simulink model "DC Dynamic Indhu Kanth"  (R2013a)
settings: Solver=ode45  StartTime=0.0  StopTime=2  RelTol=1e-3
libraries: powerlib x14, powerlib_extras x5, simulink x1
settings Model: Creator=Indhu Kanth  LastModifiedBy=Indhu Kanth

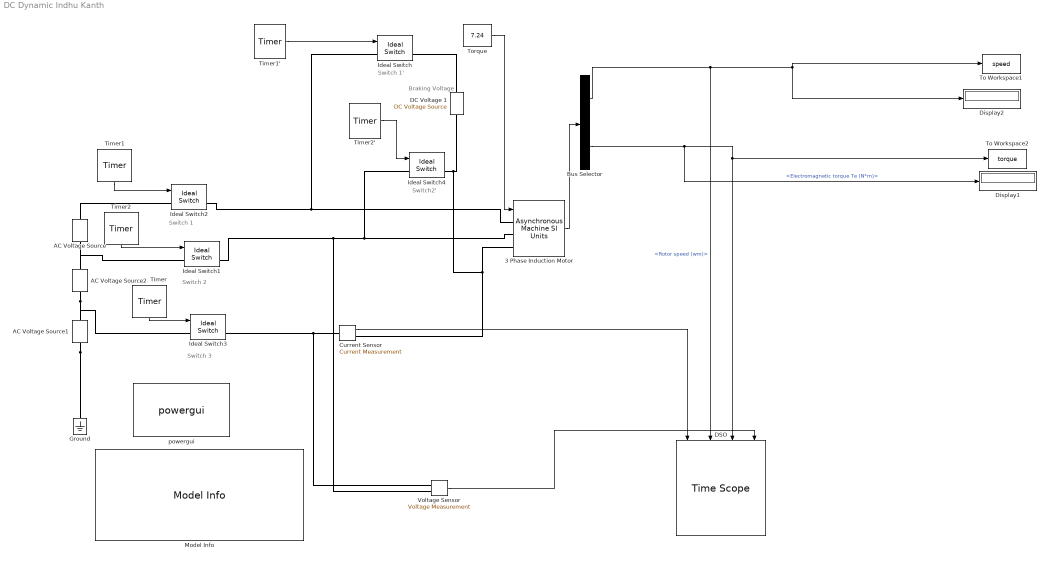
== system DC Dynamic Indhu Kanth ==
  note: Braking Voltage
  note: Switch2'
  note: Switch 1'
  note: Switch 3
  note: Switch 2
  note: Switch 1
  3 Phase Induction Motor : powerlib/Machines/Asynchronous Machine SI Units  PresetModel=No  MechanicalLoad=Torque Tm  ShowDetailedParameters=on  RotorType=Squirrel-cage  ReferenceFrame=Rotor  NominalParameters=[4427 440 50]  Stator="[0.5  0.003819]"  Rotor=[0.4 0.003819]  Cage1=[ 0.022 0.226/377]  Cage2=[ 0.022 0.226/377]  Lm=0.1591  Mechanical=[0.37 0.02791 3]  PolePairs=3  InitialConditions=[1 0 0 0 0 0 0 0]  Units=SI  LoadFlowParameters=1492000  SimulateSaturation=off  Saturation=[14.03593122, 27.81365428, 53.79336849, 72.68890987, 97.98006896, 148.6815601, 215.7428561, 302.9841135, 428.7778367 ; 230, 322, 414, 460, 506, 552, 598, 644, 690]  TsPowergui=0  TsBlock=-1  IterativeModel=Forward Euler  Pmec=0
  AC Voltage Source : powerlib/Electrical Sources/AC Voltage Source  Amplitude=230*sqrt(2)  Phase=0  Frequency=50  SampleTime=0  Measurements=None
  AC Voltage Source1 : powerlib/Electrical Sources/AC Voltage Source  Amplitude=230*sqrt(2)  Phase=120  Frequency=50  SampleTime=0  Measurements=None
  AC Voltage Source2 : powerlib/Electrical Sources/AC Voltage Source  Amplitude=230*sqrt(2)  Phase=-120  Frequency=50  SampleTime=0  Measurements=None
  Bus Selector : BusSelector  OutputSignals=Mechanical.Rotor speed (wm),Mechanical.Electromagnetic torque Te (N*m)
  Current Sensor : powerlib/Measurements/Current Measurement  PhasorSimulation=off  OutputType=Complex  PSBequivalent=0
  DC Voltage 1 : powerlib/Electrical Sources/DC Voltage Source  Amplitude=40  Measurements=None
  DSO : TimeScope  NumInputPorts=4  DefaultConfigurationName=spbscopes.TimeScopeBlockCfg
      settings: CopyFcn=scopeextensions.ScopeBlock.callback(gcbh, 'onBlockCopy', gcbh);  DeleteFcn=scopeextensions.ScopeBlock.callback(gcbh, 'onBlockDelete');  PreSaveFcn=scopeextensions.ScopeBlock.callback(gcbh, 'onModelSave');  NameChangeFcn=scopeextensions.ScopeBlock.callback(gcbh, 'onBlockRename');  CloseFcn=scopeextensions.ScopeBlock.callback(gcbh, 'onBlockClose');  PreDeleteFcn=scopeextensions.ScopeBlock.callback(gcbh, 'onBlockPreDelete');
  Display1 : Display
  Display2 : Display
  Ground : powerlib/Elements/Ground  LConnTagsString=a
  Ideal Switch : powerlib/Power Electronics/Ideal Switch  Ron=0.001  Lon=0  IC=0  Rs=1e5  Cs=inf  Measurements=on
  Ideal Switch1 : powerlib/Power Electronics/Ideal Switch  Ron=0.001  Lon=0  IC=1  Rs=1e5  Cs=inf  Measurements=on
  Ideal Switch2 : powerlib/Power Electronics/Ideal Switch  Ron=0.001  Lon=0  IC=1  Rs=1e5  Cs=inf  Measurements=on
  Ideal Switch3 : powerlib/Power Electronics/Ideal Switch  Ron=0.001  Lon=0  IC=1  Rs=1e5  Cs=inf  Measurements=on
  Ideal Switch4 : powerlib/Power Electronics/Ideal Switch  Ron=0.001  Lon=0  IC=0  Rs=1e5  Cs=inf  Measurements=on
  Model Info : simulink/Model-Wide Utilities/Model Info  InitialBlockCM=None  BlockCM=None  Frame=on  DisplayStringWithTags=|  HorizontalTextAlignment=Center  LeftAlignmentValue=0.5  SourceBlockDiagram=selfstudy1dcdynamic  TagMaxNumber=20
      | 3 PHASE INDUCTION MOTOR
      | DC Dynamic Braking
      | Indhy Kanth
  Timer : powerlib_extras/Control  Blocks/Timer  t=[0 0.5]  e="[1  0   ]"
  Timer1 : powerlib_extras/Control  Blocks/Timer  t=[0 0.5 ]  e="[1  0   ]"
  Timer1' : powerlib_extras/Control  Blocks/Timer  t=[0.5 1 ]  e=[1 1 ]
  Timer2 : powerlib_extras/Control  Blocks/Timer  t=[0 0.5 ]  e="[1  0   ]"
  Timer2' : powerlib_extras/Control  Blocks/Timer  t=[0.5 1]  e=[1 1 ]
  To Workspace1 : ToWorkspace  VariableName=speed  SampleTime=-1
  To Workspace2 : ToWorkspace  VariableName=torque  SampleTime=-1
  Torque : Constant  Value=7.24
  Voltage Sensor : powerlib/Measurements/Voltage Measurement  PhasorSimulation=off  OutputType=Complex  PSBequivalent=0
  powergui : powerlib/powergui  Priority=1  SimulationMode=Continuous  SolverType=Tustin  SampleTime=1e-6  frequency=60  SPID=off  DisableSnubberDevices=off  DisableRonSwitches=off  DisableVfSwitches=off  SwTol=0  Interpol=off  DisplayEquations=off  frequencyindice=50  Pbase=100e6  ErrMax=1e-4  Iterations=50  UnitsV=kV  UnitsW=MW  FunctionMessages=off  echomessages=off  HookPort=off  EnableUseOfTLC=off  x0status=blocks  RestoreLinks=warning  ResistiveCurrentMeasurement=off  Frange=[0:2:500]  Ylog=off  Xlog=on  ShowGrid=off  save=off  variable=ZData  ZoomFFT=on  StartTime=0.0  cycles=1  DisplayStyle=1  fundamental=60  FreqAxis=off  MaxFrequency=1000  frequencyindicesteady=1  RmsSteady=1  display=off  Ts=0  methode=off
  wires:
  Torque/1 -> 3 Phase Induction Motor/1
  Timer1/1 -> Ideal Switch2/1
  Timer2/1 -> Ideal Switch1/1
  Timer/1 -> Ideal Switch3/1
  Timer2'/1 -> Ideal Switch4/1
  Timer1'/1 -> Ideal Switch/1
  3 Phase Induction Motor/1 -> Bus Selector/1
  Bus Selector/1 -> Display2/1, To Workspace1/1, DSO/2  "<Rotor speed (wm)>"
  Bus Selector/2 -> Display1/1, To Workspace2/1, DSO/3  "<Electromagnetic torque Te (N*m)>"
  Voltage Sensor/1 -> DSO/4
  Current Sensor/1 -> DSO/1
  connections:
  AC Voltage Source2/LConn1 -- AC Voltage Source/LConn1 -- Ground/LConn1 -- AC Voltage Source1/LConn1
  Ideal Switch2/RConn1 -- Ideal Switch/LConn1 -- 3 Phase Induction Motor/LConn1
  Ideal Switch4/LConn1 -- Voltage Sensor/LConn2 -- Ideal Switch1/RConn1 -- 3 Phase Induction Motor/LConn2
  Ideal Switch1/LConn1 -- AC Voltage Source2/RConn1
  Ideal Switch2/LConn1 -- AC Voltage Source/RConn1
  AC Voltage Source1/RConn1 -- Ideal Switch3/LConn1
  3 Phase Induction Motor/LConn3 -- DC Voltage 1/LConn1 -- Ideal Switch4/RConn1 -- Current Sensor/RConn1
  DC Voltage 1/RConn1 -- Ideal Switch/RConn1
  Ideal Switch3/RConn1 -- Voltage Sensor/LConn1 -- Current Sensor/LConn1
